simulink model "simulation31"  (R2015b)
settings: Solver=VariableStepAuto  StartTime=0.0  StopTime=10.0  RelTol=1e-3
values from neighbouring files (symbols this model uses):
  A = [ ... (first row only)    [stateSpaceModel.m]
  B = [ ... (first row only)    [stateSpaceModel.m]
  C = [ ... (first row only)    [stateSpaceModel.m]
  D = [ ... (first row only)    [stateSpaceModel.m]
  Kr = -0.807    [findingKr.m]
  r_c = 5    [run_task_31.m]
  Tw = 1    [findingKr.m]
libraries: simulink_extras x3
settings Model: Creator=ShivJeet  LastModifiedBy=ShivJeet

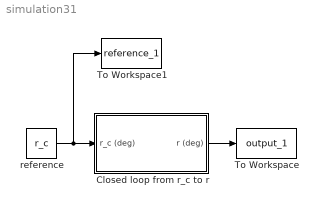
== system simulation31 ==
  Closed loop from r_c to r : Subsystem
  To Workspace : ToWorkspace  VariableName=output_1  SaveFormat=Timeseries  SampleTime=-1
  To Workspace1 : ToWorkspace  VariableName=reference_1  SaveFormat=Timeseries  SampleTime=-1
  reference : Constant  Value=r_c
  wires:
  reference/1 -> To Workspace1/1, Closed loop from r_c to r/1(r_c (deg))
  Closed loop from r_c to r/1(r (deg)) -> To Workspace/1

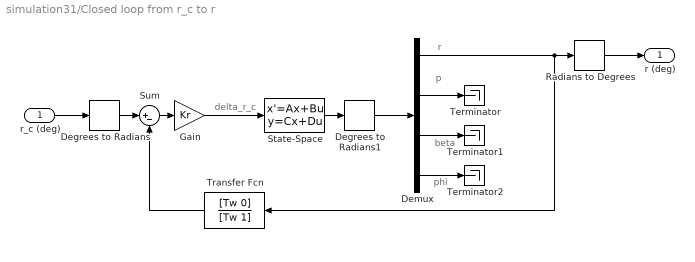
== system simulation31/Closed loop from r_c to r ==
  note: r
  note: p
  note: beta
  note: phi
  note: delta_r_c
  r_c (deg) : Inport
  Degrees to Radians : simulink_extras/Transformations/Degrees to Radians
  Degrees to Radians1 : simulink_extras/Transformations/Degrees to Radians
  Demux : Demux
  Gain : Gain  Gain=Kr
  Radians to Degrees : simulink_extras/Transformations/Radians to Degrees
  State-Space : StateSpace  A=A  B=B(:,2)  C=C  D=D(:,2)  X0=0
  Sum : Sum  Inputs=|+-
  Terminator : Terminator
  Terminator1 : Terminator
  Terminator2 : Terminator
  Transfer Fcn : TransferFcn  Numerator=[Tw 0]  Denominator=[Tw 1]
  r (deg) : Outport
  wires:
  Sum/1 -> Gain/1
  Radians to Degrees/1 -> r (deg)/1
  Demux/3 -> Terminator1/1
  Transfer Fcn/1 -> Sum/2
  Gain/1 -> State-Space/1
  r_c (deg)/1 -> Degrees to Radians/1
  Demux/4 -> Terminator2/1
  Demux/2 -> Terminator/1
  Degrees to Radians/1 -> Sum/1
  State-Space/1 -> Degrees to Radians1/1
  Demux/1 -> Radians to Degrees/1, Transfer Fcn/1
  Degrees to Radians1/1 -> Demux/1
